simulink model "force_controller_old3"  (R2024b)
settings: Solver=VariableStepAuto  StartTime=0.0  StopTime=3  RelTol=1e-3
undefined symbols (not defined in the file or in its folder): extractTop2x2, non_linear_m, non_linear_vcfg, wall_surface
libraries: roblocks x6

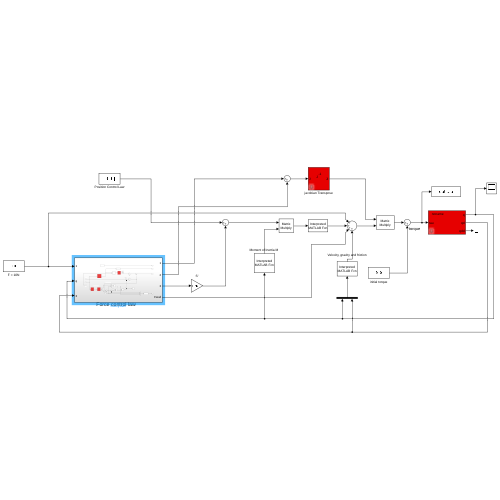
[thumbnail: Simulink's stored preview of the top-level diagram]
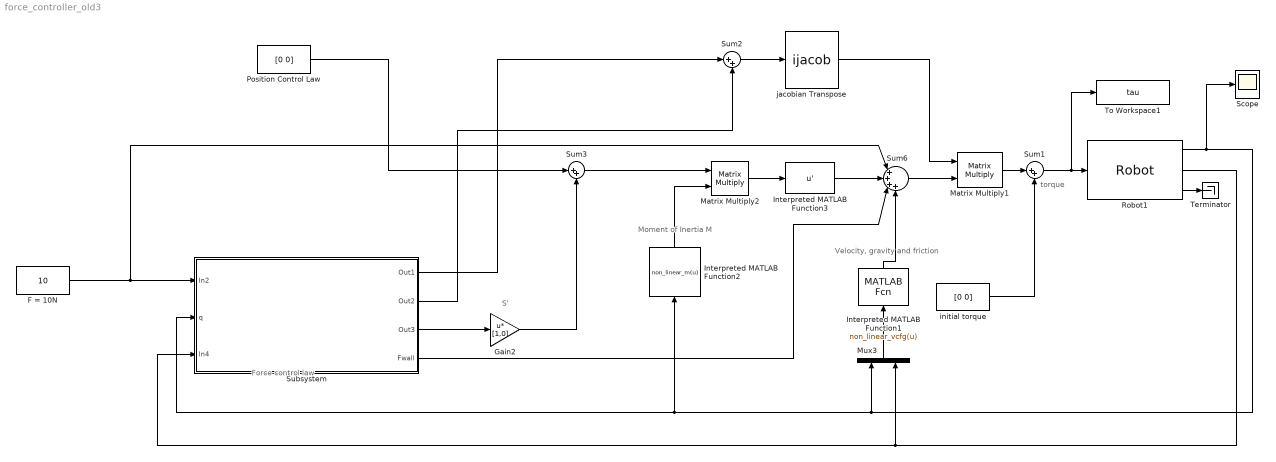
== system force_controller_old3 ==
  note: S'
  note: Force control law
  note: Moment of Inertia M
  note: Velocity, gravity and friction
  note: torque
  F = 10N : Constant  Value=10
  Gain2 : Gain  Gain=[1,0]  Multiplication=Matrix(u*K)
  Interpreted MATLAB Function1 : MATLABFcn  MATLABFcn=non_linear_vcfg(u)  OutputDimensions=[2 1]  Output1D=off
  Interpreted MATLAB Function2 : MATLABFcn  MATLABFcn=non_linear_m(u)  OutputDimensions=[2 2]  Output1D=off
  Interpreted MATLAB Function3 : MATLABFcn  MATLABFcn=u'  OutputDimensions=[2 1]  Output1D=off
  Matrix Multiply1 : Product  Multiplication=Matrix(*)
  Matrix Multiply2 : Product  Multiplication=Matrix(*)
  Mux3 : Mux  Inputs=2
  Position Control Law : Constant  Value=[0 0]
  Robot1 : roblocks/Robot  robot=robot  q0=[0 0 0 0 0 0]
      link override Integrator: InitialCondition=[1 1]
      link override Integrator1: InitialCondition=[1 1]
  Scope : Scope
  Subsystem : Subsystem
  Sum1 : Sum  Inputs=|++
  Sum2 : Sum  Inputs=|++
  Sum3 : Sum  Inputs=|++
  Sum6 : Sum  Inputs=|++++
  Terminator : Terminator
  To Workspace1 : ToWorkspace  VariableName=tau  SampleTime=-1
      settings: Save2DSignal=2-D array (concatenate along first dimension)
  initial torque : Constant  Value=[0 0]
  jacobian Transpose : roblocks/ijacob
      link override inverse jacobian: MATLABFcn=u'
  wires:
  Robot1/2 -> Subsystem/3(In4), Mux3/2
  Robot1/1 -> Scope/1, Subsystem/2(q), Interpreted MATLAB Function2/1, Mux3/1
  initial torque/1 -> Sum1/2
  Sum6/1 -> Matrix Multiply1/2
  jacobian Transpose/1 -> Matrix Multiply1/1
  Interpreted MATLAB Function2/1 -> Matrix Multiply2/2
  Matrix Multiply2/1 -> Interpreted MATLAB Function3/1
  Mux3/1 -> Interpreted MATLAB Function1/1
  Robot1/3 -> Terminator/1
  Matrix Multiply1/1 -> Sum1/1
  Sum1/1 -> Robot1/1, To Workspace1/1
  Sum2/1 -> jacobian Transpose/1
  Subsystem/1(Out1) -> Sum2/1
  Subsystem/2(Out2) -> Sum2/2
  Subsystem/3(Out3) -> Gain2/1
  Sum3/1 -> Matrix Multiply2/1
  Gain2/1 -> Sum3/2
  Position Control Law/1 -> Sum3/1
  Interpreted MATLAB Function1/1 -> Sum6/4
  Interpreted MATLAB Function3/1 -> Sum6/2
  F = 10N/1 -> Sum6/1, Subsystem/1(In2)
  Subsystem/4(Fwall) -> Sum6/3

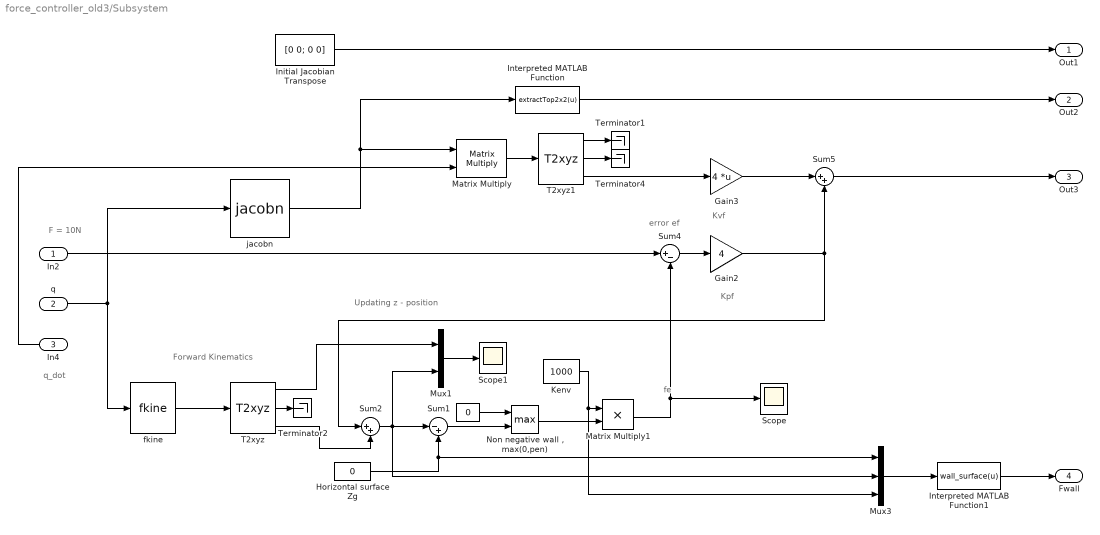
== system force_controller_old3/Subsystem ==
  note: Updating z - position
  note: Forward Kinematics
  note: F = 10N
  note: q_dot
  note: Kvf
  note: error ef
  note: Kpf
  note: fe
  In2 : Inport
  q : Inport  Port=2
  In4 : Inport  Port=3
  " " : Constant  Value=0
  " Horizontal surface Zg" : Constant  Value=0
  " Kenv" : Constant  Value=1000
  Gain2 : Gain  Gain=4
  Gain3 : Gain  Gain=4  Multiplication=Matrix(K*u)
  Initial Jacobian Transpose : Constant  Value=[0 0; 0 0]
  Interpreted MATLAB Function : MATLABFcn  MATLABFcn=extractTop2x2(u)  OutputDimensions=[2 2]  Output1D=off
  Interpreted MATLAB Function1 : MATLABFcn  MATLABFcn=wall_surface(u)  OutputDimensions=[2 1]  Output1D=off
  Matrix Multiply : Product  Multiplication=Matrix(*)
  Matrix Multiply1 : Product
  Mux1 : Mux  Inputs=2
  Mux3 : Mux  Inputs=3
  "Non negative wall , max(0,pen)" : MinMax  Function=max  Inputs=2
  Scope : Scope
  Scope1 : Scope
  Sum1 : Sum  Inputs=|-+
  Sum2 : Sum  Inputs=|++
  Sum4 : Sum  Inputs=|+-
  Sum5 : Sum  Inputs=|++
  T2xyz : roblocks/T2xyz
  T2xyz1 : roblocks/T2xyz
      link override MATLAB Fcn: MATLABFcn=transljac(u)
  Terminator1 : Terminator
  Terminator2 : Terminator
  Terminator4 : Terminator
  fkine : roblocks/fkine  robot=robot
  jacobn : roblocks/jacobn  robot=robot
      link override MATLAB Fcn: MATLABFcn=jacobn(robot,u)
  Out1 : Outport
  Out2 : Outport  Port=2
  Out3 : Outport  Port=3
  Fwall : Outport  Port=4
  wires:
  Interpreted MATLAB Function/1 -> Out2/1
  In4/1 -> Matrix Multiply/2
  Initial Jacobian Transpose/1 -> Out1/1
  Gain3/1 -> Sum5/1
  Gain2/1 -> Sum5/2, Sum2/1
  jacobn/1 -> Interpreted MATLAB Function/1, Matrix Multiply/1
  Sum5/1 -> Out3/1
  T2xyz1/3 -> Gain3/1
  q/1 -> jacobn/1, fkine/1
  Matrix Multiply/1 -> T2xyz1/1
  In2/1 -> Sum4/1
  T2xyz/2 -> Terminator2/1
  T2xyz1/1 -> Terminator1/1
  T2xyz1/2 -> Terminator4/1
  T2xyz/1 -> Mux1/1
  " Horizontal surface Zg"/1 -> Sum1/2, Mux3/1
  Sum1/1 -> "Non negative wall , max(0,pen)"/2
  " "/1 -> "Non negative wall , max(0,pen)"/1
  Sum4/1 -> Gain2/1
  " Kenv"/1 -> Mux3/3, Matrix Multiply1/1
  "Non negative wall , max(0,pen)"/1 -> Matrix Multiply1/2
  Matrix Multiply1/1 -> Sum4/2, Scope/1
  Interpreted MATLAB Function1/1 -> Fwall/1
  fkine/1 -> T2xyz/1
  T2xyz/3 -> Sum2/2
  Sum2/1 -> Mux1/2, Mux3/2, Sum1/1
  Mux3/1 -> Interpreted MATLAB Function1/1
  Mux1/1 -> Scope1/1
